simulink model "Exp3"  (R2023a)
settings: Solver=ode8  StartTime=0.0  StopTime=50  FixedStep=0.01  RelTol=1e-3
values from neighbouring files (symbols this model uses):
  A = [0 1;-k/m -b/m]    [Exp3_y_4_Val_Matrices.m]
  B = [0;1/m]    [Exp3_y_4_Val_Matrices.m]
  C = [1 0]    [Exp3_y_4_Val_Matrices.m]
  y0 = [0;0]    [Exp3_y_4_Val_Matrices.m]
settings Model: Creator=carlo  LastModifiedBy=carlo

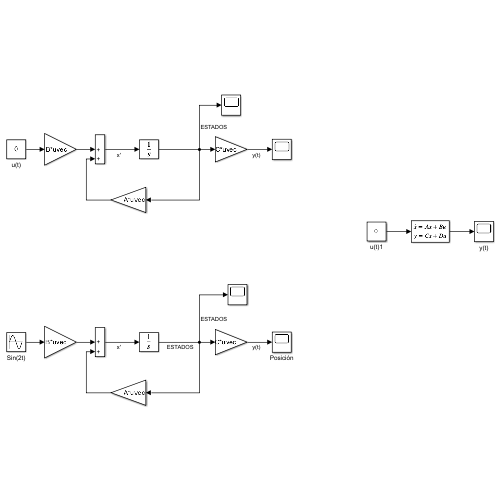
[thumbnail: Simulink's stored preview of the top-level diagram]
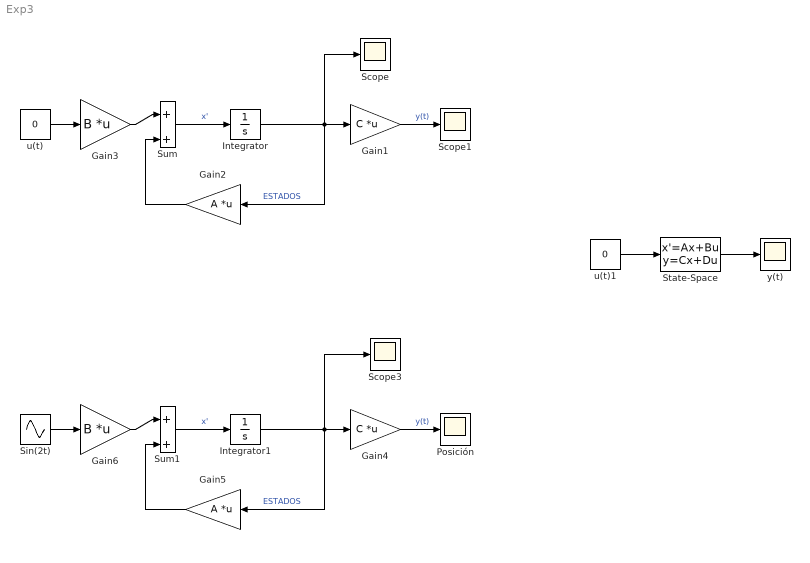
== system Exp3 ==
  Gain1 : Gain  Gain=C  Multiplication=Matrix(K*u) (u vector)
  Gain2 : Gain  Gain=A  Multiplication=Matrix(K*u) (u vector)
  Gain3 : Gain  Gain=B  Multiplication=Matrix(K*u) (u vector)
  Gain4 : Gain  Gain=C  Multiplication=Matrix(K*u) (u vector)
  Gain5 : Gain  Gain=A  Multiplication=Matrix(K*u) (u vector)
  Gain6 : Gain  Gain=B  Multiplication=Matrix(K*u) (u vector)
  Integrator : Integrator  InitialCondition=y0
  Integrator1 : Integrator  InitialCondition=y0
  Posición : Scope
  Scope : Scope
  Scope1 : Scope
  Scope3 : Scope
  Sin(2t) : Sin  Frequency=2  SampleTime=0
  State-Space : StateSpace  A=A  B=B  C=C  D=0  InitialCondition=y0
  Sum : Sum  Inputs=|++
  Sum1 : Sum  Inputs=|++
  u(t) : Constant  Value=0
  u(t)1 : Constant  Value=0
  y(t) : Scope
  wires:
  u(t)/1 -> Gain3/1
  Integrator/1 -> Scope/1, Gain2/1, Gain1/1  "ESTADOS"
  Gain2/1 -> Sum/2
  Gain3/1 -> Sum/1
  Sum/1 -> Integrator/1  "x'"
  Gain1/1 -> Scope1/1  "y(t)"
  u(t)1/1 -> State-Space/1
  State-Space/1 -> y(t)/1
  Gain5/1 -> Sum1/2
  Sum1/1 -> Integrator1/1  "x'"
  Gain4/1 -> Posición/1  "y(t)"
  Gain6/1 -> Sum1/1
  Integrator1/1 -> Scope3/1, Gain5/1, Gain4/1  "ESTADOS"
  Sin(2t)/1 -> Gain6/1
